simulink model "Type_5_Wind_Turbine_Drivetrain_Simulink_Model"  (R2019b)
settings: Solver=VariableStepAuto  StartTime=0.0  StopTime=50  MaxStep=0.005  RelTol=1e-1  AbsTol=1e-2
InitFcn:
  | Ts =2.5e-5;
  | 
  | R_pu = 0.005;
  | X_pu = 0.03;
  | B_pu = 0.00275;
  | 
  | Z_161 = 259.21;
  | Z_44 = 19.36;
  | Z_46 = 237.75;
  | Z_12_47 = 17.47;
  | 
  | AB_load_data;
  | AB_init;
values from neighbouring files (symbols this model uses):
  alpha_i_exit = deg2rad(16.21 + bias_i)    [Type_5_Torque_Converter_Initialization.m]
  alpha_i_inlet = deg2rad(-40.7 - inlet_bias_i)    [Type_5_Torque_Converter_Initialization.m]
  alpha_s_exit_0 = fzero(@(x) myfun(x),0)    [Type_5_Torque_Converter_Initialization.m]
  alpha_s_inlet = deg2rad(60.36 + inlet_bias_s)    [Type_5_Torque_Converter_Initialization.m]
  alpha_t_exit = deg2rad(-53.14 - bias_t)    [Type_5_Torque_Converter_Initialization.m]
  alpha_t_inlet = deg2rad(59.19 + inlet_bias_t)    [Type_5_Torque_Converter_Initialization.m]
  Ao = 0.0107*(pa^2)    (= 0.07974603)    [Type_5_Torque_Converter_Initialization.m]
  Cshi = 1.011    [Type_5_Torque_Converter_Initialization.m]
  Cshs = 0.773    [Type_5_Torque_Converter_Initialization.m]
  Csht = 1.8    [Type_5_Torque_Converter_Initialization.m]
  f = 0.197    [Type_5_Torque_Converter_Initialization.m]
  Ii = 0.0926    [Type_5_Torque_Converter_Initialization.m]
  It = 0.0267    [Type_5_Torque_Converter_Initialization.m]
  K4 = 35800000*(2/5)    (= 14320000)    [Type_5_Torque_Converter_Initialization.m]
  Lf = 0.2594*pa    (= 0.708162)    [Type_5_Torque_Converter_Initialization.m]
  p = 840    [Type_5_Torque_Converter_Initialization.m]
  Ri_exit = 0.0991*pa    (= 0.270543)    [Type_5_Torque_Converter_Initialization.m]
  Ri_inlet = Rs_exit    (= 0.181545)    [Type_5_Torque_Converter_Initialization.m]
  Rs_exit = 0.0665*pa    (= 0.181545)    [Type_5_Torque_Converter_Initialization.m]
  Rt_exit = 0.0735*pa    (= 0.200655)    [Type_5_Torque_Converter_Initialization.m]
  Rt_inlet = Ri_exit    (= 0.270543)    [Type_5_Torque_Converter_Initialization.m]
  Si = -1.0859e-3    (= -0.0010859)    [Type_5_Torque_Converter_Initialization.m]
  St = -2.1537e-5    (= -2.1537e-05)    [Type_5_Torque_Converter_Initialization.m]
  ti = p*Q0*(wi_0*Ri_exit^2      + V_0*(Ri_exit*tan(alpha_i_exit) - Rs_exit*tan(alpha_s_exit_0)))    [Type_5_Torque_Converter_Initialization.m]
  tt = -tgen    (= -10610.3295395)    [Type_5_Torque_Converter_Initialization.m]
  V_0 = Q0/Ao    [Type_5_Torque_Converter_Initialization.m]
  wi_0 = (1.0/nu)*wt_0    (= 188.495559215)    [Type_5_Torque_Converter_Initialization.m]
  wt_0 = (N/3600)*120*pi    (= 188.495559215)    [Type_5_Torque_Converter_Initialization.m]
undefined symbols (not defined in the file or in its folder): Tlss0
libraries: powerlib x8, simulink x1, sps_avr x1
settings Model: Creator=HUSST  LastModifiedBy=HUSST

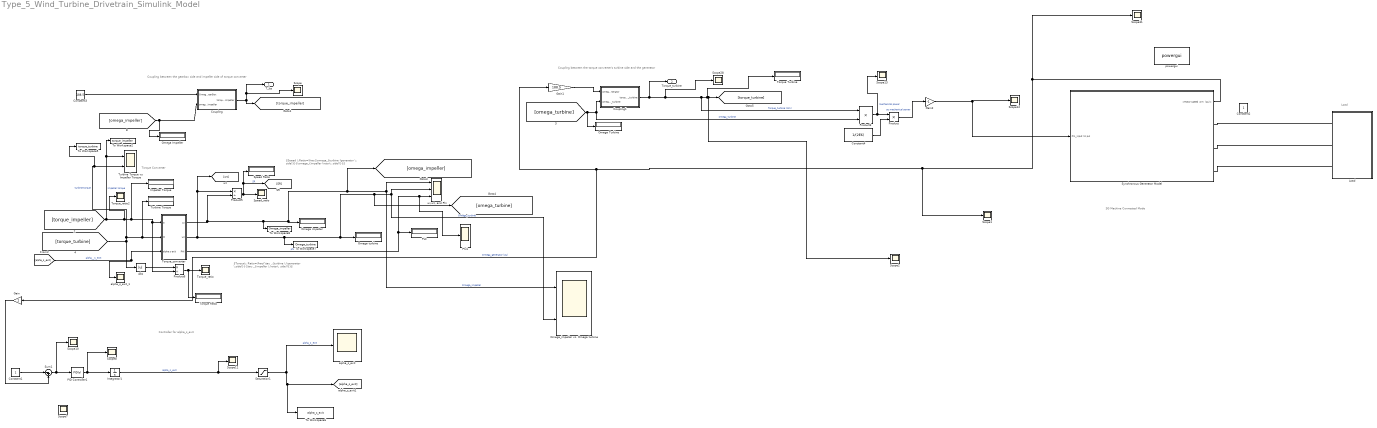
== system Type_5_Wind_Turbine_Drivetrain_Simulink_Model ==
  note: $Speed \;Ratio=\frac{\omega_{turbine (generator \; side)}}{\omega_{impeller (rotor\; side))}}$
  note: $Torque\; Ratio=\frac{\tau _{turbine \;(generator \;side)}}{\tau _{impeller \;(rotor\; side))}}$
  note: Torque Converter
  note: Coupling between the gearbox side and impeller side of torque converter
  note: Controller for alpha_s_exit
  note: Coupling between the torque converter's turbine side and the generator
  note: SG Machine Connected Mode
  note: Load
  Abs : Abs
  Constant1 : Constant
  Constant2 : Constant
  Constant3 : Constant  Value=188.5
  Constant4 : Constant  Value=1/(2E6)
  Coupling : Subsystem
  Coupling1 : Subsystem
  Gain : Gain
  Gain1 : Gain  Gain=188.5
  Gain2 : Gain  Gain=-1
  Impeller Torque : Display
  Integrator1 : Integrator  InitialCondition=alpha_s_exit_0
  "Load " : Subsystem
  Omega Impeller : Display
  Omega Turbine : Display
  Omega impeller : Display
  Omega turbine : Display
  Omega_impeller vs. Omega turbine : Scope  NumInputPorts=2
  PHI : Display
  PID Controller1 : simulink/Continuous/PID Controller  Controller=PID  Form=Parallel  TimeDomain=Continuous-time  SampleTime=-1  IntegratorMethod=Forward Euler  FilterMethod=Forward Euler  ControllerParametersSource=internal  P=8  I=1  D=10  UseFilter=on  N=100  TunerSelectOption=Transfer Function Based (PID Tuner App)  InitialConditionSource=internal  InitialConditionForIntegrator=0  InitialConditionForFilter=0  DifferentiatorICPrevScaledInput=0  ExternalReset=none  TrackingMode=off  Kt=1  LimitOutput=off  UpperSaturationLimit=inf  LowerSaturationLimit=-inf  LinearizeAsGain=on  AntiWindupMode=none  Kb=1  POutMin=[]  POutMax=[]  IOutMin=[]  IOutMax=[]  DOutMin=[]  DOutMax=[]  NOutMin=[]  NOutMax=[]  SumOutMin=[]  SumOutMax=[]  SaturationOutMin=[]  SaturationOutMax=[]  PParamMin=[]  PParamMax=[]  IParamMin=[]  IParamMax=[]  DParamMin=[]  DParamMax=[]  NParamMin=[]  NParamMax=[]  KbParamMin=[]  KbParamMax=[]  KtParamMin=[]  KtParamMax=[]  KbOutMin=[]  KbOutMax=[]  KtOutMin=[]  KtOutMax=[]  IntegratorOutMin=[]  IntegratorOutMax=[]  FilterOutMin=[]  FilterOutMax=[]  SumI1OutMin=[]  SumI1OutMax=[]  SumI2OutMin=[]  SumI2OutMax=[]  SumI3OutMin=[]  SumI3OutMax=[]  SumI4OutMin=[]  SumI4OutMax=[]  SumDOutMin=[]  SumDOutMax=[]  DifferentiatorOutMin=[]  DifferentiatorOutMax=[]  FilterDiffOutCoefMin=[]  FilterDiffOutCoefMax=[]  ReciprocalOutMin=[]  ReciprocalOutMax=[]  SumDenOutMin=[]  SumDenOutMax=[]  SumNumOutMin=[]  SumNumOutMax=[]  DivideOutMin=[]  DivideOutMax=[]  IntegratorContinuousStateAttributes=''  IntegratorStateMustResolveToSignalObject=off  IntegratorRTWStateStorageClass=Auto  FilterContinuousStateAttributes=''  FilterStateMustResolveToSignalObject=off  FilterRTWStateStorageClass=Auto  ParallelPVariant=InternalParameters  IdealPVariant=Disabled  IVariant=InternalParameters  DVariant=InternalParameters  IntegratorVariant=Continuous  SatVariant=Disabled  AWVariant=Passthrough  PCopyVariant=Disabled  TRVariant=Disabled  FdbkBlocksVariant=Forward  IdealPFdbkVariant=Disabled  SatFdbkVariant=Disabled  DerivativeFilterVariant=ContFilter  NVariant=InternalParameters  NCopyVariant=Disabled  FilterICVariant=InternalICsFilter  IntegratorICVariant=InternalICs  ExternalResetVariant=Disabled  TRSumVariant=Passthrough  SumFdbkVariant=Disabled  SumVariant=Sum_PID
  Phi1 : Scope
  Product : Product
  Product3 : Product  Inputs=**
  Product5 : Product  Inputs=*/
  Product6 : Product  Inputs=*/
  Saturation1 : Saturate  UpperLimit=1.28  LowerLimit=1.04
  Scope{,1..2,7..8,10..13,28,31} (11 alike) : Scope
  Speed Ratio : Display
  Speed_ratio : Scope
  Sum1 : Sum  Inputs=|-+
  Synchronous Generator Model : Subsystem
  To Workspace2 : ToWorkspace  VariableName=torque_impeller  SampleTime=1e-2
  To Workspace5 : ToWorkspace  VariableName=torque_turbine  SampleTime=1e-2
  To Workspace6 : ToWorkspace  VariableName=alpha_s_exit  SampleTime=1e-2
  To Workspace7 : ToWorkspace  VariableName=Omega_turbine  SampleTime=1e-2
  To Workspace8 : ToWorkspace  VariableName=Omega_impeller  SampleTime=1e-2
  Torque Ratio : Display
  Torque Turbine : Display
  Torque_converter : Subsystem
  Torque_ratio : Scope
  Torque_ratio2 : Scope
  Turbine Torque : Display
  Turbine Torque vs Impeller Torque : Scope  NumInputPorts=2
  alpha_s_exit : Scope
  alpha_s_exit_1 : Scope
  powergui : powerlib/powergui  Priority=1  SimulationMode=Discrete  SampleTime=Ts  frequency=60  Iterations=50  frequencyindice=60  Pbase=8.9e6  ErrMax=0.0001  UnitsV=kV  UnitsW=MW  buscounter=0  FunctionMessages=off  echomessages=off  EnableUseOfTLC=off  CurrentSourceSwitches=off  DisableSnubberDevices=off  DisableRonSwitches=off  DisableVfSwitches=off  DisplayEquations=off  AutomaticDiscreteSolvers=off  SolverType=Tustin/Backward Euler (TBE)  Interpol=off  ExternalGateDelay=off  methode=off  Ts=100  x0status=blocks  SPID=on  SwTol=0  HookPort=off  NonlinearTolerance=1e-4  nMaxIteration=100  ContinueOnMaxIteration=off  RestoreLinks=warning  ResistiveCurrentMeasurement=off  Frange=[0:2:500]  Ylog=off  Xlog=on  ShowGrid=off  save=off  variable=ZData  structure=0  ZoomFFT=off  StartTime=0.0  cycles=1  DisplayStyle=1  fundamental=60  FreqAxis=off  MaxFrequency=1000  frequencyindicesteady=1  RmsSteady=1  display=off
      settings: SourceProductName=Simscape Electrical
  "wi,wt, and Phi" : Scope  NumInputPorts=3
  T_lss : Outport  InitialOutput=Tlss0
  Torque_turbine : Outport  Port=2  InitialOutput=Tlss0
  wires:
  Product6/1 -> Torque_ratio/1, Torque Ratio/1
  Torque_converter/2(wt) -> Product5/1, [wt], To Workspace7/1, [omega_turbine], Omega_impeller vs. Omega turbine/2, "wi,wt, and Phi"/2, Omega turbine/1  "Omega_turbine"
  Torque_converter/1(wi) -> Product5/2, To Workspace8/1, Omega impeller/1, [omega_impeller], Omega_impeller vs. Omega turbine/1, "wi,wt, and Phi"/1  "Omega_impeller"
  Product5/1 -> [SR], Speed Ratio/1, Speed_ratio/1  "SR"
  Torque_converter/3(PHI) -> Phi1/1, "wi,wt, and Phi"/3, PHI/1  "phi"
  Abs/1 -> Product6/1
  [torque_turbine] -> To Workspace5/1, Turbine Torque vs Impeller Torque/2, Turbine Torque/1, Torque_converter/2(tt), Abs/1  "turbine torque"
  [alpha_s_exit] -> Torque_converter/3(alpha s exit), alpha_s_exit_1/1  "alpha__s_exit"
  [torque_impeller] -> Torque_ratio2/1, Impeller Torque/1, Product6/2, Torque_converter/1(ti), To Workspace2/1, Turbine Torque vs Impeller Torque/1  "impeller torque"
  Constant3/1 -> Coupling/1(Omega_gearBox)
  [omega_impeller] -> Omega Impeller/1, Coupling/2(omega_impeller)
  Coupling/1(torque_impeller) -> T_lss/1, Scope/1, [torque_impeller]
  Integrator1/1 -> Saturation1/1, Scope11/1  "alpha_s_exit"
  Saturation1/1 -> To Workspace6/1, [alpha_s_exit], alpha_s_exit/1  "alpha_s_exit"
  Sum1/1 -> Scope10/1, PID Controller1/1
  PID Controller1/1 -> Integrator1/1, Scope8/1
  Constant1/1 -> Sum1/1
  Gain/1 -> Sum1/2
  Product3/1 -> Scope13/1, Product/1  "mechanical power"
  Gain1/1 -> Coupling1/1(omega_generator)
  Coupling1/1(torque_turbine) -> Torque_turbine/1, Scope28/1, Product3/1, Torque Turbine/1, Scope2/1, [torque_turbine]  "Torque_turbine (Nm)"
  Constant4/1 -> Product/2
  [omega_turbine] -> Omega Turbine/1, Coupling1/2(omega_turbine), Product3/2  "omega_turbine"
  Product/1 -> Gain2/1  "pu mechanical power"
  Synchronous Generator Model/1(<Rotor speed  wm  (pu)>) -> Scope31/1, Scope1/1, Gain/1, Gain1/1  "Omega_generator (pu)"
  Gain2/1 -> Scope12/1, Synchronous Generator Model/1(Pm_input (in pu))
  connections:
  Synchronous Generator Model/RConn3 -- "Load "/LConn3
  Synchronous Generator Model/RConn1 -- "Load "/LConn1
  Synchronous Generator Model/RConn2 -- "Load "/LConn2

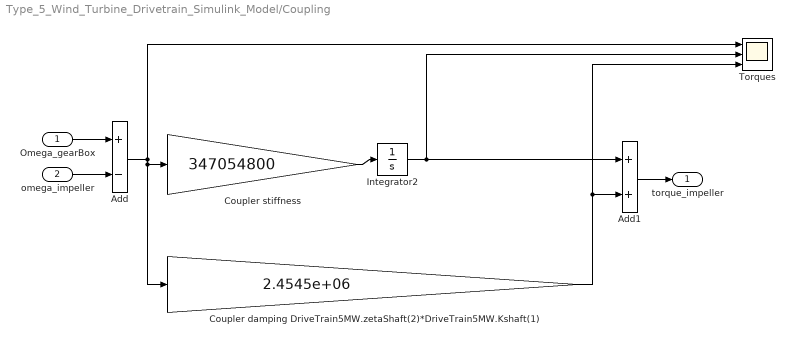
== system Type_5_Wind_Turbine_Drivetrain_Simulink_Model/Coupling ==
  Omega_gearBox : Inport
  omega_impeller : Inport  Port=2
  Add : Sum  Inputs=+-
  Add1 : Sum
  "Coupler damping DriveTrain5MW.zetaShaft(2)*DriveTrain5MW.Kshaft(1) " : Gain  Gain=2.4545e+06
  Coupler stiffness : Gain  Gain=347054800
  Integrator2 : Integrator  InitialCondition=ti  ContinuousStateAttributes='torquelowspeedshaft'
  Torques : Scope  NumInputPorts=3
  torque_impeller : Outport
  wires:
  "Coupler damping DriveTrain5MW.zetaShaft(2)*DriveTrain5MW.Kshaft(1) "/1 -> Add1/2, Torques/3
  Add1/1 -> torque_impeller/1
  Integrator2/1 -> Add1/1, Torques/2
  Omega_gearBox/1 -> Add/1
  omega_impeller/1 -> Add/2
  Add/1 -> Coupler stiffness/1, "Coupler damping DriveTrain5MW.zetaShaft(2)*DriveTrain5MW.Kshaft(1) "/1, Torques/1
  Coupler stiffness/1 -> Integrator2/1

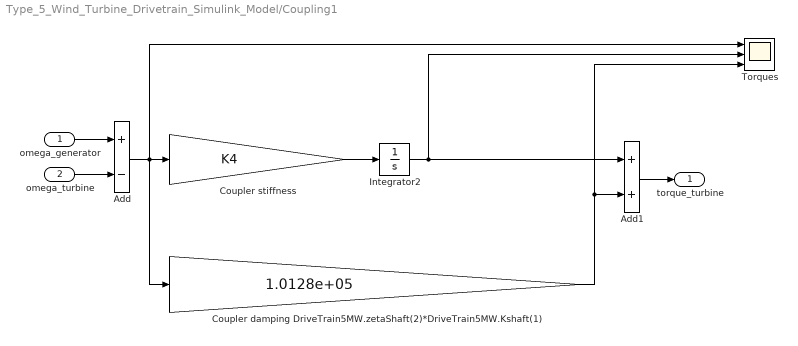
== system Type_5_Wind_Turbine_Drivetrain_Simulink_Model/Coupling1 ==
  omega_generator : Inport
  omega_turbine : Inport  Port=2
  Add : Sum  Inputs=+-
  Add1 : Sum
  "Coupler damping DriveTrain5MW.zetaShaft(2)*DriveTrain5MW.Kshaft(1) " : Gain  Gain=1.0128e+05
  Coupler stiffness : Gain  Gain=K4
  Integrator2 : Integrator  InitialCondition=tt  ContinuousStateAttributes='torquelowspeedshaft'
  Torques : Scope  NumInputPorts=3
  torque_turbine : Outport
  wires:
  "Coupler damping DriveTrain5MW.zetaShaft(2)*DriveTrain5MW.Kshaft(1) "/1 -> Add1/2, Torques/3
  Add1/1 -> torque_turbine/1
  Integrator2/1 -> Add1/1, Torques/2
  omega_generator/1 -> Add/1
  omega_turbine/1 -> Add/2
  Add/1 -> Coupler stiffness/1, Torques/1, "Coupler damping DriveTrain5MW.zetaShaft(2)*DriveTrain5MW.Kshaft(1) "/1
  Coupler stiffness/1 -> Integrator2/1

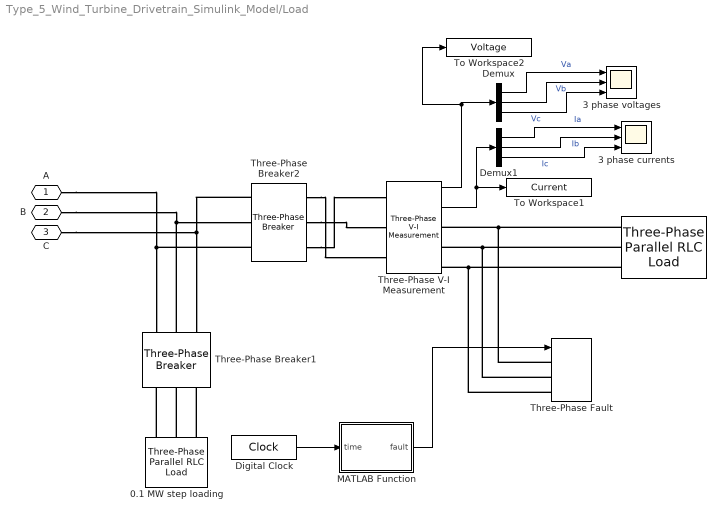
== system Type_5_Wind_Turbine_Drivetrain_Simulink_Model/Load  ==
  "  " : powerlib/Elements/Three-Phase Parallel RLC Load  LConnTagsString=A|B|C  Configuration=Y (grounded)  NominalVoltage=4.16e3  Vabc=[1e3 1e3 1e3]  Vabcp=[1e3 1e3 1e3]  NominalFrequency=60  UnbalancedPower=off  ActivePower=1.9E6  InductivePower=0  CapacitivePower=0  Pabc=[10e3 9e3 11e3]  QLabc=[100 90 110]  QCabc=[100 90 110]  Pabcp=[10e3 9e3 11e3]  QLabcp=[100 90 110]  QCabcp=[100 90 110]  Measurements=None  LoadType=constant Z
  0.1 MW step loading : powerlib/Elements/Three-Phase Parallel RLC Load  LConnTagsString=A|B|C  Configuration=Y (grounded)  NominalVoltage=4.16e3  Vabc=[1e3 1e3 1e3]  Vabcp=[1e3 1e3 1e3]  NominalFrequency=60  UnbalancedPower=off  ActivePower=.4E6  InductivePower=0  CapacitivePower=0  Pabc=[10e3 9e3 11e3]  QLabc=[100 90 110]  QCabc=[100 90 110]  Pabcp=[10e3 9e3 11e3]  QLabcp=[100 90 110]  QCabcp=[100 90 110]  Measurements=None  LoadType=constant Z
  3 phase currents : Scope  NumInputPorts=3
  3 phase voltages : Scope  NumInputPorts=3
  Demux : Demux  Outputs=3
  Demux1 : Demux  Outputs=3
  Digital Clock : DigitalClock  SampleTime=Ts
  MATLAB Function : MATLAB Function  TreatAsAtomicUnit=on
  Three-Phase V-I Measurement : powerlib/Measurements/Three-Phase V-I Measurement  VoltageMeasurement=phase-to-ground  SetLabelV=off  LabelV=Vabc  Vpu=off  VpuLL=off  CurrentMeasurement=yes  SetLabelI=off  LabelI=Iabc  Ipu=off  Pbase=100e6  Vbase=500e3  OutputType=Complex  PhasorSimulation=off  PSBequivalent=0
      settings: SourceProductName=Simscape Electrical
  Three-Phase Breaker1 : powerlib/Elements/Three-Phase Breaker  InitialState=open  SwitchA=on  SwitchB=on  SwitchC=on  SwitchTimes=[460]  External=off  BreakerResistance=0.0001  SnubberResistance=1e10  SnubberCapacitance=inf  Measurements=None
  Three-Phase Breaker2 : powerlib/Elements/Three-Phase Breaker  InitialState=closed  SwitchA=on  SwitchB=on  SwitchC=on  SwitchTimes=[150]  External=off  BreakerResistance=0.0001  SnubberResistance=1e10  SnubberCapacitance=inf  Measurements=None
  Three-Phase Fault : powerlib/Elements/Three-Phase Fault  InitialStates=0  FaultA=on  FaultB=on  FaultC=on  GroundFault=on  SwitchTimes="[1/60  5/60]"  External=on  SwitchStatus=NaN  FaultResistance=0.001  GroundResistance=0.01  SnubberResistance=1e6  SnubberCapacitance=inf  Measurements=None
      settings: SourceProductName=Simscape Electrical
  To Workspace1 : ToWorkspace  VariableName=Current  SampleTime=-1
  To Workspace2 : ToWorkspace  VariableName=Voltage  SampleTime=-1
  A : PMIOPort  Side=Left
  B : PMIOPort  Port=2  Side=Left
  C : PMIOPort  Port=3  Side=Left
  wires:
  Digital Clock/1 -> MATLAB Function/1(time)
  MATLAB Function/1(fault) -> Three-Phase Fault/1
  Three-Phase V-I Measurement/1 -> To Workspace2/1, Demux/1
  Three-Phase V-I Measurement/2 -> Demux1/1, To Workspace1/1
  Demux/1 -> 3 phase voltages/1  "Va"
  Demux/2 -> 3 phase voltages/2  "Vb"
  Demux/3 -> 3 phase voltages/3  "Vc"
  Demux1/3 -> 3 phase currents/3  "Ic"
  Demux1/1 -> 3 phase currents/1  "Ia"
  Demux1/2 -> 3 phase currents/2  "Ib"
  connections:
  Three-Phase Breaker1/RConn2 -- B/RConn1 -- Three-Phase Breaker2/RConn2
  A/RConn1 -- Three-Phase Breaker2/RConn1 -- Three-Phase Breaker1/RConn1
  C/RConn1 -- Three-Phase Breaker1/RConn3 -- Three-Phase Breaker2/RConn3
  0.1 MW step loading/LConn2 -- Three-Phase Breaker1/LConn2
  0.1 MW step loading/LConn3 -- Three-Phase Breaker1/LConn3
  0.1 MW step loading/LConn1 -- Three-Phase Breaker1/LConn1
  Three-Phase Breaker2/LConn1 -- Three-Phase V-I Measurement/LConn1
  Three-Phase Breaker2/LConn2 -- Three-Phase V-I Measurement/LConn2
  Three-Phase Breaker2/LConn3 -- Three-Phase V-I Measurement/LConn3
  "  "/LConn1 -- Three-Phase Fault/LConn1 -- Three-Phase V-I Measurement/RConn1
  "  "/LConn2 -- Three-Phase Fault/LConn2 -- Three-Phase V-I Measurement/RConn2
  "  "/LConn3 -- Three-Phase Fault/LConn3 -- Three-Phase V-I Measurement/RConn3

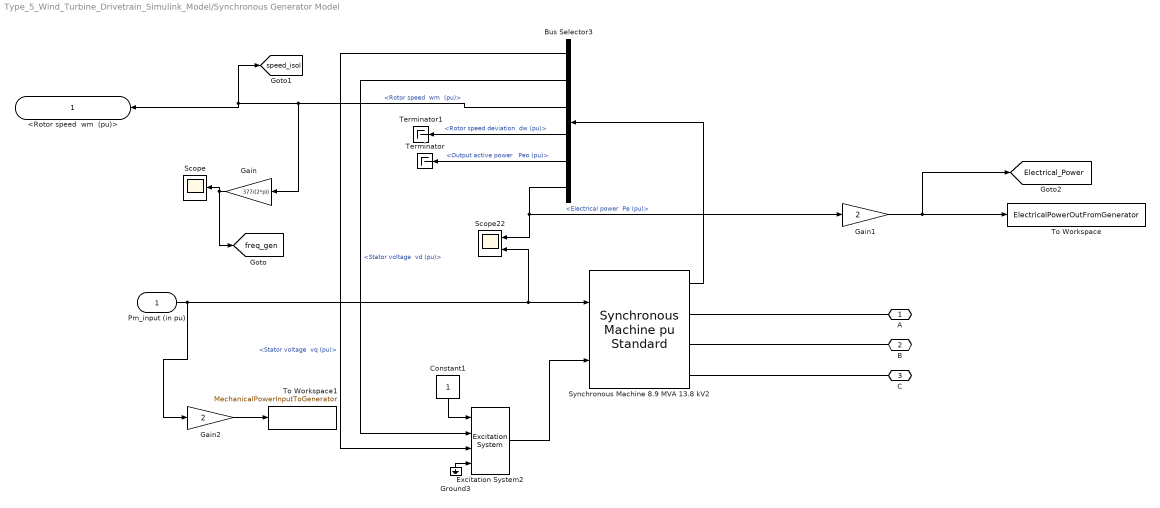
== system Type_5_Wind_Turbine_Drivetrain_Simulink_Model/Synchronous Generator Model ==
  Pm_input (in pu) : Inport
  Bus Selector3 : BusSelector  OutputSignals="dq0 components.Stator voltage  vq (pu),dq0 components.Stator voltage  vd (pu),Mechanical.Rotor speed  wm  (pu),Mechanical.Rotor speed deviation  dw (pu),Output active power   Peo (pu),Mechanical.Electrical power  Pe (pu)"
  Constant1 : Constant
  Excitation System2 : sps_avr/Excitation System  tr=20e-3  reg=[ 300, 0.01 ]  exc=[ 1, 0 ]  tgr=[ 0, 0 ]  damp=[ 0.001, 0.1 ]  sat=[ 0, 0 ]  lim=[-2.5, 2.5, 0 ]  v0=[1,1.02102]
      settings: SourceProductBaseCode=PS
  Gain : Gain  Gain=377/(2*pi)
  Gain1 : Gain  Gain=2
  Gain2 : Gain  Gain=2
  Ground3 : Ground
  Scope : Scope
  Scope22 : Scope  NumInputPorts=2
  Synchronous Machine 8.9 MVA 13.8 kV2 : powerlib/Machines/Synchronous Machine pu Standard  PresetModel=No  MechanicalLoad=Mechanical power Pm  ShowDetailedParameters=on  RotorType=Salient-pole  Units=per unit standard parameters  MeasurementBus=off  NominalParameters="[ 2E6  4160   60 ]"  Reactances1=[ 31 32 33 34 35 36 37 ]  Reactances2=[ 0.85, 0.35, 0.30, 0.5, 0.36, 0.18 ]  dAxisTimeConstants=Short-circuit  qAxisTimeConstants=Open-circuit  TimeConstants1=[]  TimeConstants2=[]  TimeConstants3=[]  TimeConstants4=[]  TimeConstants5=[ 0.7, 0.053, 0.1 ]  TimeConstants6=[]  TimeConstants7=[]  TimeConstants8=[]  StatorResistance=2.8544e-3  Mechanical=[1.33 0 2]  PolePairs=2  InitialConditions=[0 -82.5714 0.260966 0.260966 0.260966 0 -120 120 1.02102]  SetSaturation=off  Saturation=[0.6404,0.7127,0.8441,0.9214,0.9956,1.082,1.19,1.316,1.457;0.7,0.7698,0.8872,0.9466,0.9969,1.046,1.1,1.151,1.201]  LoadFlowParameters=[2 154000000 0 0]  TsPowergui=0  TsBlock=-1  IterativeModel=Trapezoidal non iterative  IterativeDiscreteModel=Trapezoidal non iterative  BusType=swing  Pref=2e6  Qref=0  Qmin=-Inf  Qmax=Inf  PLF=0  QLF=0
      settings: AttributesFormatString=\n\n
  Terminator : Terminator
  Terminator1 : Terminator
  To Workspace : ToWorkspace  VariableName=ElectricalPowerOutFromGenerator  SaveFormat=Timeseries  SampleTime=1e-2
  To Workspace1 : ToWorkspace  VariableName=MechanicalPowerInputToGenerator  SaveFormat=Timeseries  SampleTime=-1
  A : PMIOPort  Side=Right
  B : PMIOPort  Port=2  Side=Right
  C : PMIOPort  Port=3  Side=Right
  <Rotor speed  wm  (pu)> : Outport
  tag scope: Electrical_Power=global, freq_gen=global, speed_isol=global
  wires:
  Bus Selector3/6 -> Scope22/1, Gain1/1  "<Electrical power  Pe (pu)>"
  Bus Selector3/2 -> Excitation System2/2  "<Stator voltage  vd (pu)>"
  Ground3/1 -> Excitation System2/4
  Bus Selector3/1 -> Excitation System2/3  "<Stator voltage  vq (pu)>"
  Excitation System2/1 -> Synchronous Machine 8.9 MVA 13.8 kV2/2
  Constant1/1 -> Excitation System2/1
  Synchronous Machine 8.9 MVA 13.8 kV2/1 -> Bus Selector3/1
  Bus Selector3/3 -> Gain/1, [speed_isol], <Rotor speed  wm  (pu)>/1  "<Rotor speed  wm  (pu)>"
  Pm_input (in pu)/1 -> Gain2/1, Synchronous Machine 8.9 MVA 13.8 kV2/1, Scope22/2
  Bus Selector3/4 -> Terminator1/1  "<Rotor speed deviation  dw (pu)>"
  Bus Selector3/5 -> Terminator/1  "<Output active power   Peo (pu)>"
  Gain/1 -> Scope/1, [freq_gen]
  Gain2/1 -> To Workspace1/1
  Gain1/1 -> [Electrical_Power], To Workspace/1
  connections:
  Synchronous Machine 8.9 MVA 13.8 kV2/RConn3 -- C/RConn1
  Synchronous Machine 8.9 MVA 13.8 kV2/RConn1 -- A/RConn1
  Synchronous Machine 8.9 MVA 13.8 kV2/RConn2 -- B/RConn1

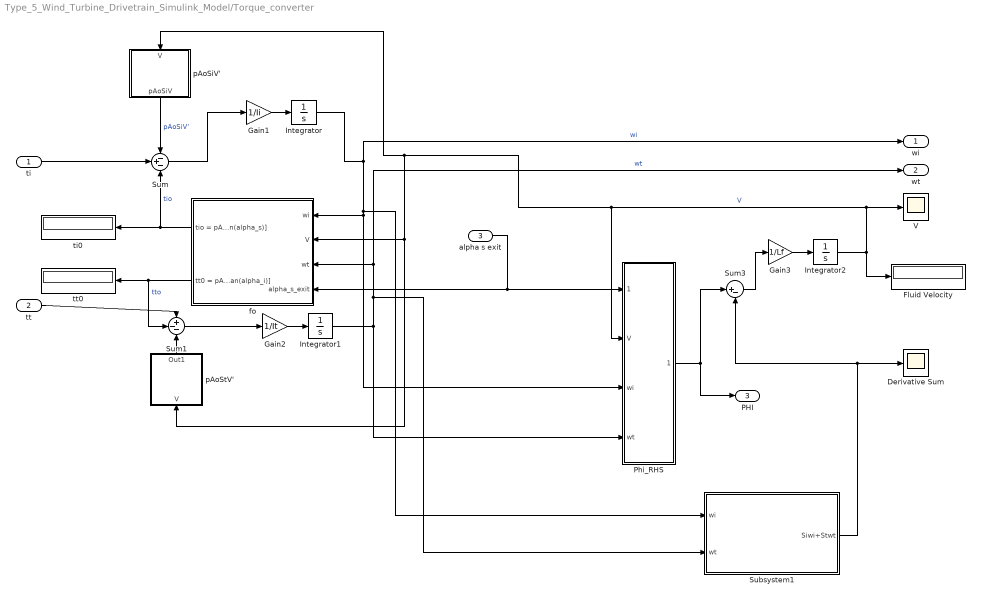
== system Type_5_Wind_Turbine_Drivetrain_Simulink_Model/Torque_converter ==
  ti : Inport
  tt : Inport  Port=2
  alpha s exit : Inport  Port=3
  Derivative Sum : Scope
  Fluid Velocity : Display
  Gain1 : Gain  Gain=1/Ii
  Gain2 : Gain  Gain=1/It
  Gain3 : Gain  Gain=1/Lf
  Integrator : Integrator  InitialCondition=wi_0
  Integrator1 : Integrator  InitialCondition=wt_0
  Integrator2 : Integrator  InitialCondition=V_0
  Phi_RHS : Subsystem
  Subsystem1 : Subsystem
  Sum : Sum  Inputs=-+-
  Sum1 : Sum  Inputs=+--
  Sum3 : Sum  Inputs=|+-
  V : Scope
  fo : Subsystem
  pAoSiV' : Subsystem
  pAoStV' : Subsystem
  ti0 : Display
  tt0 : Display
  wi : Outport
  wt : Outport  Port=2
  PHI : Outport  Port=3
  wires:
  Integrator2/1 -> Fluid Velocity/1, V/1, Phi_RHS/2(V), pAoStV'/1(V), fo/2(V), pAoSiV'/1(V)  "V"
  fo/1(tio = pAoV[wi*Ri^2 + V*Ri*tan(alpha_i) - ws*Rs^2 - V*Rs*tan(alpha_s)]) -> ti0/1, Sum/3  "tio"
  fo/2(tt0 = pAoV[wt*Rt^2 + V*Rt*tan(alpha_t) - wi*Ri^2 - V*Ri*tan(alpha_i)]) -> tt0/1, Sum1/2  "tto"
  Sum3/1 -> Gain3/1
  tt/1 -> Sum1/1
  Subsystem1/1(Siwi+Stwt) -> Sum3/2, Derivative Sum/1
  pAoSiV'/1(pAoSiV) -> Sum/1  "pAoSiV'"
  pAoStV'/1(Out1) -> Sum1/3
  Sum1/1 -> Gain2/1
  ti/1 -> Sum/2
  Integrator/1 -> Phi_RHS/3(wi), fo/1(wi), Subsystem1/1(wi), wi/1  "wi"
  Integrator1/1 -> Phi_RHS/4(wt), wt/1, fo/3(wt), Subsystem1/2(wt)  "wt"
  Sum/1 -> Gain1/1
  Gain1/1 -> Integrator/1
  Gain2/1 -> Integrator1/1
  Gain3/1 -> Integrator2/1
  alpha s exit/1 -> Phi_RHS/1(alpha_s_exit), fo/4(alpha_s_exit)
  Phi_RHS/1(Phi_RHS) -> PHI/1, Sum3/1

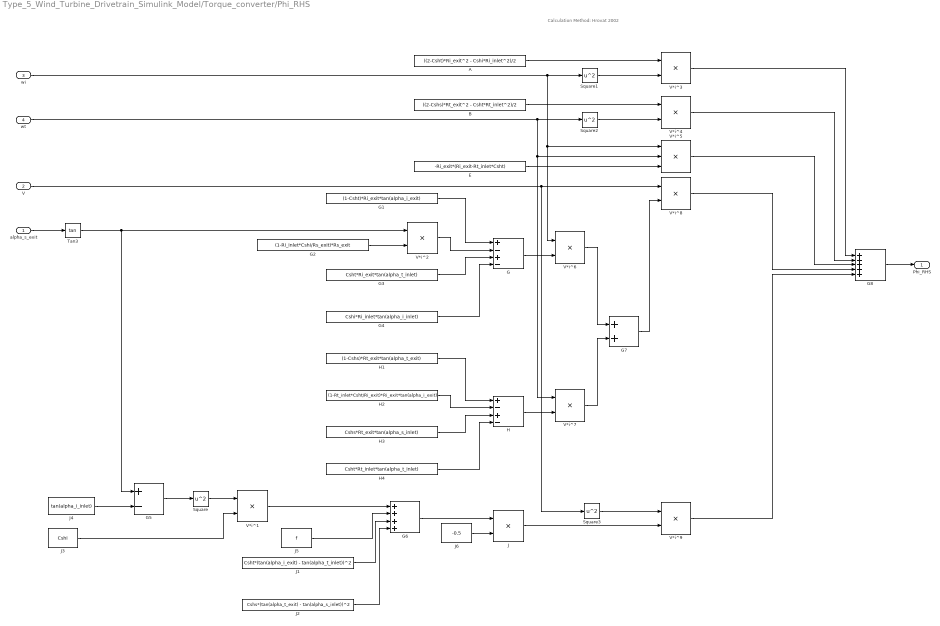
== system Type_5_Wind_Turbine_Drivetrain_Simulink_Model/Torque_converter/Phi_RHS ==
  note: Calculation Method: Hrovat 2002
  alpha_s_exit : Inport
  V : Inport  Port=2
  wi : Inport  Port=3
  wt : Inport  Port=4
  A : Constant  Value=((2-Csht)*Ri_exit^2 - Cshi*Ri_inlet^2)/2
  B : Constant  Value=((2-Cshs)*Rt_exit^2 - Csht*Rt_inlet^2)/2
  E : Constant  Value=-Ri_exit*(Ri_exit-Rt_inlet*Csht)
  G : Sum  Inputs=+-+-
  G1 : Constant  Value=(1-Csht)*Ri_exit*tan(alpha_i_exit)
  G2 : Constant  Value=(1-Ri_inlet*Cshi/Rs_exit)*Rs_exit
  G3 : Constant  Value=Csht*Ri_exit*tan(alpha_t_inlet)
  G4 : Constant  Value=Cshi*Ri_inlet*tan(alpha_i_inlet)
  G5 : Sum  Inputs=+-
  G6 : Sum  Inputs=++++
  G7 : Sum
  G8 : Sum  Inputs=+++++
  H : Sum  Inputs=+-+-
  H1 : Constant  Value=(1-Cshs)*Rt_exit*tan(alpha_t_exit)
  H2 : Constant  Value=(1-Rt_inlet*Csht/Ri_exit)*Ri_exit*tan(alpha_i_exit)
  H3 : Constant  Value=Cshs*Rt_exit*tan(alpha_s_inlet)
  H4 : Constant  Value=Csht*Rt_inlet*tan(alpha_t_inlet)
  J : Product
  J1 : Constant  Value=Csht*(tan(alpha_i_exit) - tan(alpha_t_inlet))^2
  J2 : Constant  Value=Cshs*(tan(alpha_t_exit) - tan(alpha_s_inlet))^2
  J3 : Constant  Value=Cshi
  J4 : Constant  Value=tan(alpha_i_inlet)
  J5 : Constant  Value=f
  J6 : Constant  Value=-0.5
  Square{,1..3} (4 alike) : Math  Operator=square  SignedPower=off  SaturateOnIntegerOverflow=on
  Tan3 : Trigonometry  Operator=tan
  V*i^{1..4,6..9} (8 alike) : Product
  V*i^5 : Product  Inputs=3
  Phi_RHS : Outport
  wires:
  alpha_s_exit/1 -> Tan3/1
  G2/1 -> V*i^2/2
  Tan3/1 -> G5/1, V*i^2/1
  G1/1 -> G/1
  V*i^2/1 -> G/2
  G3/1 -> G/3
  G4/1 -> G/4
  H1/1 -> H/1
  H2/1 -> H/2
  H3/1 -> H/3
  H4/1 -> H/4
  J3/1 -> V*i^1/2
  J4/1 -> G5/2
  G5/1 -> Square/1
  Square/1 -> V*i^1/1
  V*i^1/1 -> G6/1
  J5/1 -> G6/2
  J1/1 -> G6/3
  J2/1 -> G6/4
  G6/1 -> J/1
  J6/1 -> J/2
  A/1 -> V*i^3/1
  wi/1 -> V*i^5/1, V*i^6/1, Square1/1
  Square1/1 -> V*i^3/2
  B/1 -> V*i^4/1
  Square2/1 -> V*i^4/2
  wt/1 -> V*i^7/1, V*i^5/2, Square2/1
  E/1 -> V*i^5/3
  G/1 -> V*i^6/2
  H/1 -> V*i^7/2
  V*i^6/1 -> G7/1
  V*i^7/1 -> G7/2
  V/1 -> V*i^8/1, Square3/1
  G7/1 -> V*i^8/2
  J/1 -> V*i^9/2
  Square3/1 -> V*i^9/1
  V*i^9/1 -> G8/5
  V*i^8/1 -> G8/4
  V*i^5/1 -> G8/3
  V*i^4/1 -> G8/2
  V*i^3/1 -> G8/1
  G8/1 -> Phi_RHS/1

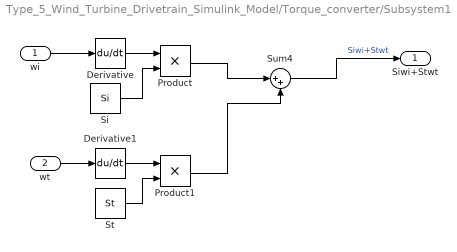
== system Type_5_Wind_Turbine_Drivetrain_Simulink_Model/Torque_converter/Subsystem1 ==
  wi : Inport
  wt : Inport  Port=2
  Derivative : Derivative  CoefficientInTFapproximation=0
  Derivative1 : Derivative  CoefficientInTFapproximation=0
  Product : Product
  Product1 : Product
  Si : Constant  Value=Si
  St : Constant  Value=St
  Sum4 : Sum  Inputs=|++
  Siwi+Stwt : Outport
  wires:
  Derivative1/1 -> Product1/1
  Product1/1 -> Sum4/2
  Si/1 -> Product/2
  Product/1 -> Sum4/1
  St/1 -> Product1/2
  Derivative/1 -> Product/1
  wt/1 -> Derivative1/1
  wi/1 -> Derivative/1
  Sum4/1 -> Siwi+Stwt/1  "Siwi+Stwt"

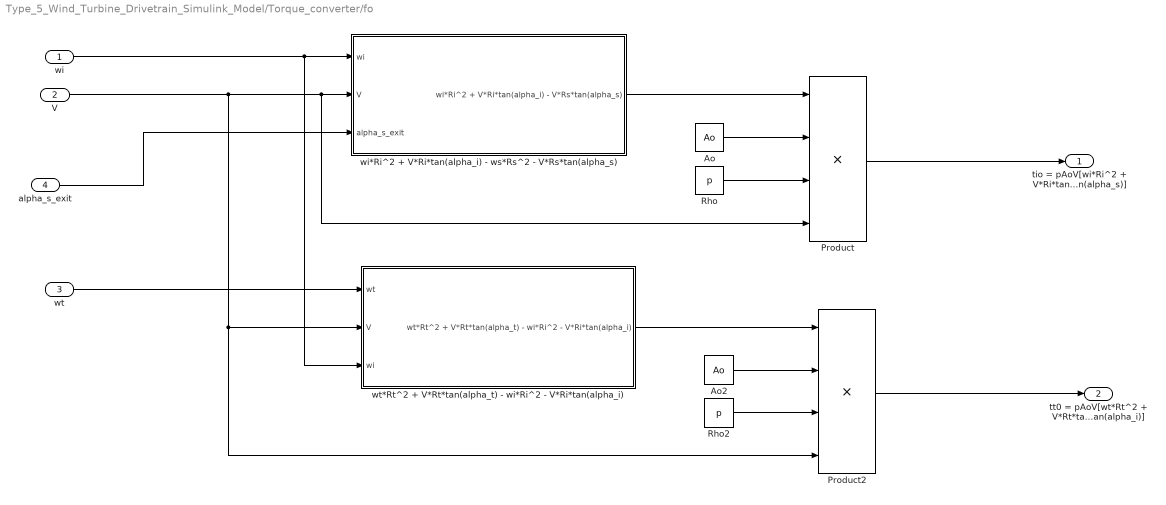
== system Type_5_Wind_Turbine_Drivetrain_Simulink_Model/Torque_converter/fo ==
  wi : Inport
  V : Inport  Port=2
  wt : Inport  Port=3
  alpha_s_exit : Inport  Port=4
  Ao : Constant  Value=Ao
  Ao2 : Constant  Value=Ao
  Product : Product  Inputs=4
  Product2 : Product  Inputs=4
  Rho : Constant  Value=p
  Rho2 : Constant  Value=p
  "wi*Ri^2 + V*Ri*tan(alpha_i) - ws*Rs^2 - V*Rs*tan(alpha_s)   " : Subsystem
  "wt*Rt^2 + V*Rt*tan(alpha_t) - wi*Ri^2 - V*Ri*tan(alpha_i)   " : Subsystem
  tio = pAoV[wi*Ri^2 + V*Ri*tan(alpha_i) - ws*Rs^2 - V*Rs*tan(alpha_s)] : Outport
  tt0 = pAoV[wt*Rt^2 + V*Rt*tan(alpha_t) - wi*Ri^2 - V*Ri*tan(alpha_i)] : Outport  Port=2
  wires:
  Rho2/1 -> Product2/3
  Ao/1 -> Product/2
  Product2/1 -> tt0 = pAoV[wt*Rt^2 + V*Rt*tan(alpha_t) - wi*Ri^2 - V*Ri*tan(alpha_i)]/1
  "wt*Rt^2 + V*Rt*tan(alpha_t) - wi*Ri^2 - V*Ri*tan(alpha_i)   "/1("wt*Rt^2 + V*Rt*tan(alpha_t) - wi*Ri^2 - V*Ri*tan(alpha_i)   ") -> Product2/1
  "wi*Ri^2 + V*Ri*tan(alpha_i) - ws*Rs^2 - V*Rs*tan(alpha_s)   "/1("wi*Ri^2 + V*Ri*tan(alpha_i) - V*Rs*tan(alpha_s)   ") -> Product/1
  Ao2/1 -> Product2/2
  wi/1 -> "wt*Rt^2 + V*Rt*tan(alpha_t) - wi*Ri^2 - V*Ri*tan(alpha_i)   "/3(wi), "wi*Ri^2 + V*Ri*tan(alpha_i) - ws*Rs^2 - V*Rs*tan(alpha_s)   "/1(wi)
  Rho/1 -> Product/3
  wt/1 -> "wt*Rt^2 + V*Rt*tan(alpha_t) - wi*Ri^2 - V*Ri*tan(alpha_i)   "/1(wt)
  V/1 -> Product/4, "wi*Ri^2 + V*Ri*tan(alpha_i) - ws*Rs^2 - V*Rs*tan(alpha_s)   "/2(V), "wt*Rt^2 + V*Rt*tan(alpha_t) - wi*Ri^2 - V*Ri*tan(alpha_i)   "/2(V), Product2/4
  Product/1 -> tio = pAoV[wi*Ri^2 + V*Ri*tan(alpha_i) - ws*Rs^2 - V*Rs*tan(alpha_s)]/1
  alpha_s_exit/1 -> "wi*Ri^2 + V*Ri*tan(alpha_i) - ws*Rs^2 - V*Rs*tan(alpha_s)   "/3(alpha_s_exit)

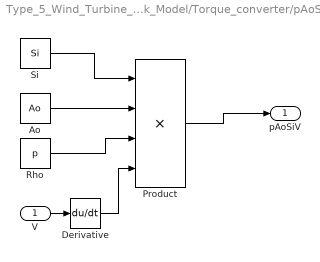
== system Type_5_Wind_Turbine_Drivetrain_Simulink_Model/Torque_converter/pAoSiV' ==
  V : Inport
  Ao : Constant  Value=Ao
  Derivative : Derivative  CoefficientInTFapproximation=0
  Product : Product  Inputs=4
  Rho : Constant  Value=p
  Si : Constant  Value=Si
  pAoSiV : Outport
  wires:
  Rho/1 -> Product/3
  Product/1 -> pAoSiV/1
  Ao/1 -> Product/2
  Si/1 -> Product/1
  V/1 -> Derivative/1
  Derivative/1 -> Product/4

== system Type_5_Wind_Turbine_Drivetrain_Simulink_Model/Torque_converter/pAoStV' ==
  V : Inport
  Ao : Constant  Value=Ao
  Derivative : Derivative  CoefficientInTFapproximation=0
  Product : Product  Inputs=4
  Rho : Constant  Value=p
  St : Constant  Value=St
  Out1 : Outport
  wires:
  Rho/1 -> Product/3
  Product/1 -> Out1/1
  Ao/1 -> Product/2
  St/1 -> Product/1
  V/1 -> Derivative/1
  Derivative/1 -> Product/4

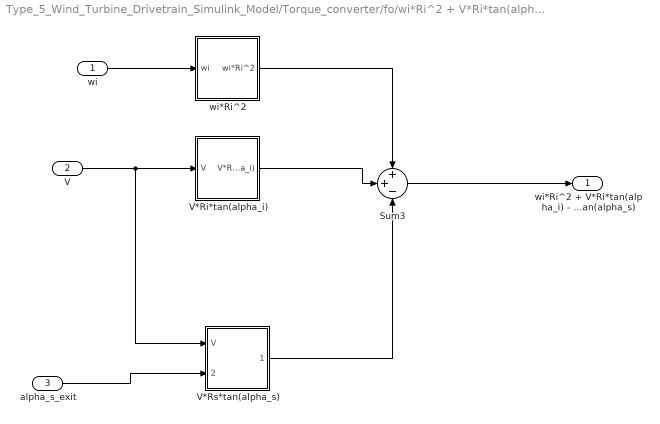
== system Type_5_Wind_Turbine_Drivetrain_Simulink_Model/Torque_converter/fo/wi*Ri^2 + V*Ri*tan(alpha_i) - ws*Rs^2 - V*Rs*tan(alpha_s)    ==
  wi : Inport
  V : Inport  Port=2
  alpha_s_exit : Inport  Port=3
  Sum3 : Sum  Inputs=++-
  V*Ri*tan(alpha_i) : Subsystem
  V*Rs*tan(alpha_s) : Subsystem
  wi*Ri^2 : Subsystem
  "wi*Ri^2 + V*Ri*tan(alpha_i) - V*Rs*tan(alpha_s)   " : Outport
  wires:
  Sum3/1 -> "wi*Ri^2 + V*Ri*tan(alpha_i) - V*Rs*tan(alpha_s)   "/1
  V*Ri*tan(alpha_i)/1(V*Ri * tan(alpha_i)) -> Sum3/2
  wi*Ri^2/1(wi*Ri^2) -> Sum3/1
  wi/1 -> wi*Ri^2/1(wi)
  V/1 -> V*Rs*tan(alpha_s)/1(V), V*Ri*tan(alpha_i)/1(V)
  V*Rs*tan(alpha_s)/1(V*Rs * tan(alpha_s)) -> Sum3/3
  alpha_s_exit/1 -> V*Rs*tan(alpha_s)/2(alpha_s_exit)

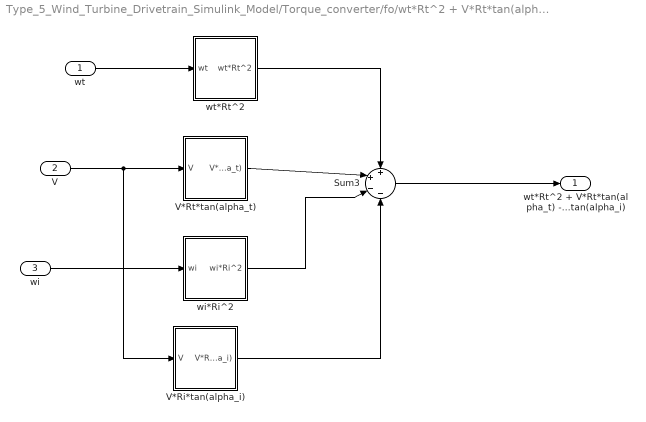
== system Type_5_Wind_Turbine_Drivetrain_Simulink_Model/Torque_converter/fo/wt*Rt^2 + V*Rt*tan(alpha_t) - wi*Ri^2 - V*Ri*tan(alpha_i)    ==
  wt : Inport
  V : Inport  Port=2
  wi : Inport  Port=3
  Sum3 : Sum  Inputs=++--
  V*Ri*tan(alpha_i) : Subsystem
  V*Rt*tan(alpha_t) : Subsystem
  wi*Ri^2 : Subsystem
  wt*Rt^2 : Subsystem
  "wt*Rt^2 + V*Rt*tan(alpha_t) - wi*Ri^2 - V*Ri*tan(alpha_i)   " : Outport
  wires:
  Sum3/1 -> "wt*Rt^2 + V*Rt*tan(alpha_t) - wi*Ri^2 - V*Ri*tan(alpha_i)   "/1
  V*Rt*tan(alpha_t)/1(V*Rt * tan(alpha_t)) -> Sum3/2
  wt*Rt^2/1(wt*Rt^2) -> Sum3/1
  wt/1 -> wt*Rt^2/1(wt)
  V/1 -> V*Ri*tan(alpha_i)/1(V), V*Rt*tan(alpha_t)/1(V)
  wi/1 -> wi*Ri^2/1(wi)
  wi*Ri^2/1(wi*Ri^2) -> Sum3/3
  V*Ri*tan(alpha_i)/1(V*Ri * tan(alpha_i)) -> Sum3/4

== system Type_5_Wind_Turbine_Drivetrain_Simulink_Model/Torque_converter/fo/wi*Ri^2 + V*Ri*tan(alpha_i) - ws*Rs^2 - V*Rs*tan(alpha_s)   /V*Ri*tan(alpha_i) ==
  V : Inport
  Product1 : Product
  Ri * tan(alpha_i) : Constant  Value=Ri_exit* tan(alpha_i_exit)
  V*Ri * tan(alpha_i) : Outport
  wires:
  Ri * tan(alpha_i)/1 -> Product1/1
  Product1/1 -> V*Ri * tan(alpha_i)/1
  V/1 -> Product1/2

== system Type_5_Wind_Turbine_Drivetrain_Simulink_Model/Torque_converter/fo/wi*Ri^2 + V*Ri*tan(alpha_i) - ws*Rs^2 - V*Rs*tan(alpha_s)   /V*Rs*tan(alpha_s) ==
  V : Inport
  alpha_s_exit : Inport  Port=2
  Product1 : Product  Inputs=3
  Rs * tan(alpha_s) : Constant  Value=Rs_exit
  Tan : Trigonometry  Operator=tan
  V*Rs * tan(alpha_s) : Outport
  wires:
  Rs * tan(alpha_s)/1 -> Product1/2
  Product1/1 -> V*Rs * tan(alpha_s)/1
  V/1 -> Product1/3
  alpha_s_exit/1 -> Tan/1
  Tan/1 -> Product1/1

== system Type_5_Wind_Turbine_Drivetrain_Simulink_Model/Torque_converter/fo/wi*Ri^2 + V*Ri*tan(alpha_i) - ws*Rs^2 - V*Rs*tan(alpha_s)   /wi*Ri^2 ==
  wi : Inport
  Product1 : Product
  Ri^2 : Constant  Value=Ri_exit^2
  wi*Ri^2 : Outport
  wires:
  Ri^2/1 -> Product1/1
  Product1/1 -> wi*Ri^2/1
  wi/1 -> Product1/2

== system Type_5_Wind_Turbine_Drivetrain_Simulink_Model/Torque_converter/fo/wt*Rt^2 + V*Rt*tan(alpha_t) - wi*Ri^2 - V*Ri*tan(alpha_i)   /V*Ri*tan(alpha_i) ==
  V : Inport
  Product1 : Product
  Ri * tan(alpha_i) : Constant  Value=Ri_exit* tan(alpha_i_exit)
  V*Ri * tan(alpha_i) : Outport
  wires:
  Ri * tan(alpha_i)/1 -> Product1/1
  Product1/1 -> V*Ri * tan(alpha_i)/1
  V/1 -> Product1/2

== system Type_5_Wind_Turbine_Drivetrain_Simulink_Model/Torque_converter/fo/wt*Rt^2 + V*Rt*tan(alpha_t) - wi*Ri^2 - V*Ri*tan(alpha_i)   /V*Rt*tan(alpha_t) ==
  V : Inport
  Product1 : Product
  Rt * tan(alpha_t) : Constant  Value=Rt_exit* tan(alpha_t_exit)
  V*Rt * tan(alpha_t) : Outport
  wires:
  Rt * tan(alpha_t)/1 -> Product1/1
  Product1/1 -> V*Rt * tan(alpha_t)/1
  V/1 -> Product1/2

== system Type_5_Wind_Turbine_Drivetrain_Simulink_Model/Torque_converter/fo/wt*Rt^2 + V*Rt*tan(alpha_t) - wi*Ri^2 - V*Ri*tan(alpha_i)   /wi*Ri^2 ==
  wi : Inport
  Product1 : Product
  Ri^2 : Constant  Value=Ri_exit^2
  wi*Ri^2 : Outport
  wires:
  Ri^2/1 -> Product1/1
  Product1/1 -> wi*Ri^2/1
  wi/1 -> Product1/2

== system Type_5_Wind_Turbine_Drivetrain_Simulink_Model/Torque_converter/fo/wt*Rt^2 + V*Rt*tan(alpha_t) - wi*Ri^2 - V*Ri*tan(alpha_i)   /wt*Rt^2 ==
  wt : Inport
  Product1 : Product
  Rt^2 : Constant  Value=Rt_exit^2
  wt*Rt^2 : Outport
  wires:
  Rt^2/1 -> Product1/1
  Product1/1 -> wt*Rt^2/1
  wt/1 -> Product1/2

== matlab function Type_5_Wind_Turbine_Drivetrain_Simulink_Model/Load /MATLAB Function ==
  data: time input; fault output
function fault = fcn(time)
fault=0;
if(time>=25 && time<=25.1) % fault cleared in 5 cycles 
    fault =1;
end
